simulink model "PIL_NO_RPI_new"  (R2021a)
settings: Solver=FixedStepAuto  StartTime=0.0  StopTime=60  FixedStep=0.001  RelTol=1e-3  EnableMultiTasking=on
values from neighbouring files (symbols this model uses):
  den_lpf_d = den_lpf20    [Mainframe_init.m]    (also in load_autopilot.m)
  Enable_Gyros = 0    [Mainframe_init.m]
  Enable_INS = 0    [Mainframe_init.m]
  num_lpf_d = num_lpf20    [Mainframe_init.m]    (also in load_autopilot.m)
undefined symbols (not defined in the file or in its folder): act_dmp, act_omega, Actuator, Aerodynamics, aMode, Autopilot, AUX, c_b_WGS, c_be, c_flat, c_grav, c_h_geop0, c_h_geope, c_pa0, c_pe, c_r0, c_rot, c_rsma, c_Tmp0, d_siB_0, d_siB_max, d_siB_min, dd_siB_max, dd_siB_min, dev, DiscIntNeverNeededParam, e_pa, e_Tmp, fin_maxrate, flag_I_act_switch, flag_I_aero_switch, flag_I_flat, flag_I_gravity_switch, flag_I_rot, h_bkpts_m, hcr, HIL_Data, JMMM_0, JMMM_e, JSPB_e, Ki_phi_vec, Kp_p_vec, Kp_phi_vec, lat_0, lon_0, Mass_Props, mB_0, mM_0, mM_e, National_Instruments, Newton, p, pBII_0, PCIe, phi, pMPB, pNPB, propellant_kg, prp_FBPB, prp_mdot ... (+40)
libraries: simulink x32, simulink_extras x23, aerolibcommonsys x4, pil_lib x2, custom_blocks x1, px4lib x1, sldrtlib x1, aerolibnav x1
(part 3 of 16)

== system PIL_NO_RPI_new/Non-linear Flight Dynamic Model1/Subsystem1/Extract States ==
  airfr_bus : Inport
  Assemble_States_Bus1 : Subsystem
  Bus Selector1 : BusSelector  OutputSignals=flight_dyn_bus.vBIB,flight_dyn_bus.wBIB,flight_dyn_bus.aBIB,flight_dyn_bus.d_wBIB,flight_dyn_bus.qIB,flight_dyn_bus.pBII,flight_dyn_bus.vBII
  MATLAB Function1 : MATLAB Function  TreatAsAtomicUnit=on
  quaternion_to_euler_angles1 : Subsystem
      mask help: transforms quaternions to Euler angles (roll, pitch, yaw)
      mask Help:
      | Name:
      | 
      |     quaternion_to_euler_angles
      | 
      | Description:
      | 
      |     This block implements the transformation of a quaternion into the
      |     corresponding Euler angles (zyx-sequence, roll, pitch, yaw).
      | 
      | Inputs  [size] [data type] [unit]:
      | 
      |     quaternion  [4] [double] [-]
      | 
      | Outputs  [size] [data type] [unit]:
      | 
      |     roll angle phi  [1] [double] [rad]
      |     pitch angle theta  [1] [double] [rad]
      |     yaw angle psi  [1] [double] [rad]
      mask Display:
      | %disp (' q --> (Phi,Theta,Psi) [rad]')
      | disp('q \rightarrow eu(\Phi;\Theta;\Psi)','texmode','on')
  States : Outport
  wires:
  Bus Selector1/6 -> Assemble_States_Bus1/6(POS_NED)  "<pBII>"
  quaternion_to_euler_angles1/1(eulx) -> Assemble_States_Bus1/5(Attitude_States)  "from Quat"
  MATLAB Function1/1(q_conj) -> quaternion_to_euler_angles1/1(q)
  Bus Selector1/5 -> MATLAB Function1/1(q)  "<qIB>"
  airfr_bus/1 -> Bus Selector1/1
  Bus Selector1/1 -> Assemble_States_Bus1/1(Translation_States)  "<vBIB>"
  Bus Selector1/2 -> Assemble_States_Bus1/2(Rotation_States)  "<wBIB>"
  Bus Selector1/4 -> Assemble_States_Bus1/4(Rotation_States_Dot)  "<d_wBIB>"
  Bus Selector1/3 -> Assemble_States_Bus1/3(Translation_States_Dot)  "<aBIB>"
  Assemble_States_Bus1/1(States) -> States/1
  Bus Selector1/7 -> Assemble_States_Bus1/7(POS_NED_dot)  "<vBII>"

== system PIL_NO_RPI_new/Non-linear Flight Dynamic Model1/Subsystem1/Fin Deflections ==
  Servo Deflections : Inport
  Add : Sum
  Bus Selector : BusSelector  OutputSignals=Fin_1,Fin_2,Fin_3,Fin_4
  Constant1 : Constant  Value=unc_fin_def_roll
  Constant2 : Constant  Value=unc_fin_def_pitch
  Constant3 : Constant  Value=unc_fin_def_yaw
  Degrees to Radians : Subsystem  mask(DegreesToRadians){}
      mask help: SimulinkBlocks:simulink_extras:DegreesToRadians_MD
      mask Help: web([docroot '/simulink/ref_extras/degreestoradians.html'])
      mask Display: disp('D2R')
  Degrees to Radians1 : Subsystem  mask(DegreesToRadians){}
      mask help: SimulinkBlocks:simulink_extras:DegreesToRadians_MD
      mask Help: web([docroot '/simulink/ref_extras/degreestoradians.html'])
      mask Display: disp('D2R')
  Degrees to Radians2 : Subsystem  mask(DegreesToRadians){}
      mask help: SimulinkBlocks:simulink_extras:DegreesToRadians_MD
      mask Help: web([docroot '/simulink/ref_extras/degreestoradians.html'])
      mask Display: disp('D2R')
  Vector Concatenate : Concatenate  NumInputs=4
  Vector Concatenate1 : Concatenate  NumInputs=3
  control_allocation : Subsystem
  afinB : Outport
  wires:
  Degrees to Radians2/1(Radians out) -> Vector Concatenate1/3
  Vector Concatenate1/1 -> control_allocation/1(fin_cmd)  "fin_cmd"
  Constant1/1 -> Degrees to Radians/1(Degrees in)  "xi_cmd"
  Degrees to Radians1/1(Radians out) -> Vector Concatenate1/2
  Degrees to Radians/1(Radians out) -> Vector Concatenate1/1
  Constant3/1 -> Degrees to Radians2/1(Degrees in)  "ze_cmd"
  Constant2/1 -> Degrees to Radians1/1(Degrees in)  "et_cmd"
  Bus Selector/2 -> Vector Concatenate/2  "<Fin_2>"
  Servo Deflections/1 -> Bus Selector/1
  Bus Selector/1 -> Vector Concatenate/1  "<Fin_1>"
  Bus Selector/4 -> Vector Concatenate/4  "<Fin_4>"
  Vector Concatenate/1 -> Add/1
  Bus Selector/3 -> Vector Concatenate/3  "<Fin_3>"
  control_allocation/1(siB_cmd) -> Add/2
  Add/1 -> afinB/1  "siB_cmd"

== system PIL_NO_RPI_new/Non-linear Flight Dynamic Model1/Subsystem1/GRM_Airframe ==
  siB_cmd : Inport
  T_sim_glbl : Inport  Port=2
  Bus Creator : BusCreator  Inputs=9
  aerodynamics : Subsystem
  environment : Subsystem
  fin_actuators : Subsystem
  forces_moments : Subsystem
  gravity : Subsystem
  input : Subsystem
  motion_kinematics : Subsystem
  propulsion : Subsystem
  rb_eom : Subsystem
  stream_flow : Subsystem
  weight_and_balance : Subsystem
  airfr : Outport  VectorParamsAs1DForOutWhenUnconnected=off
  wires:
  forces_moments/1(for_mom_bus) -> rb_eom/2(for_mom)
  [env] -> Bus Creator/9
  [fin] -> Bus Creator/7
  [motion_kin] -> Bus Creator/6
  [env_glbl] -> aerodynamics/4(env_glbl)
  aerodynamics/1(aero) -> forces_moments/1(aero), [aero]
  [motion_kin] -> rb_eom/1(mot_kin)
  weight_and_balance/1(wab) -> rb_eom/3(wab), gravity/2(wab), [wab], propulsion/2(wab)
  [wab] -> aerodynamics/3(wab)
  [str_flow] -> Bus Creator/5
  [motion_kin] -> forces_moments/2(motion_kin)
  motion_kinematics/1(motion_kin) -> stream_flow/2(motion_kin), [motion_kin]
  [grav] -> Bus Creator/3
  Bus Creator/1 -> airfr/1  "airfr_bus"
  [aero] -> Bus Creator/4
  environment/1(env) -> [env], stream_flow/3(env), gravity/1(env)
  [prp] -> forces_moments/4(prp)
  [prp] -> Bus Creator/8
  stream_flow/1(str_flow) -> [str_flow], aerodynamics/1(str_flow)
  input/1(cmd_bus) -> fin_actuators/1(cmd)
  [wab] -> Bus Creator/2
  gravity/1(grav) -> [grav], forces_moments/3(grav)
  T_sim_glbl/1 -> [env_glbl], environment/2(env_glbl), weight_and_balance/1(env_glb), propulsion/1(env_glbl)
  siB_cmd/1 -> input/1(siB_cmd)
  rb_eom/1(flight_dyn) -> environment/1(flight_dyn), motion_kinematics/1(flight_dyn), stream_flow/1(flight_dyn), Bus Creator/1
  fin_actuators/1(fin) -> [fin], aerodynamics/2(fin)
  propulsion/1(prp) -> [prp]

== system PIL_NO_RPI_new/Non-linear Flight Dynamic Model1/Translate Fins/Degrees to Radians ==
  Degrees in : Inport
  Gain1 : Gain  Gain=pi/180  SaturateOnIntegerOverflow=on  OutDataTypeStr=Inherit: Same as input  ParamDataTypeStr=Inherit: Same as input
  Radians out : Outport  InitialOutput=0  VectorParamsAs1DForOutWhenUnconnected=off
  wires:
  Gain1/1 -> Radians out/1
  Degrees in/1 -> Gain1/1

== system PIL_NO_RPI_new/Non-linear Flight Dynamic Model1/Translate Fins/Degrees to Radians1 ==
  Degrees in : Inport
  Gain1 : Gain  Gain=pi/180  SaturateOnIntegerOverflow=on  OutDataTypeStr=Inherit: Same as input  ParamDataTypeStr=Inherit: Same as input
  Radians out : Outport  InitialOutput=0  VectorParamsAs1DForOutWhenUnconnected=off
  wires:
  Gain1/1 -> Radians out/1
  Degrees in/1 -> Gain1/1

== system PIL_NO_RPI_new/Non-linear Flight Dynamic Model1/Translate Fins/Degrees to Radians2 ==
  Degrees in : Inport
  Gain1 : Gain  Gain=pi/180  SaturateOnIntegerOverflow=on  OutDataTypeStr=Inherit: Same as input  ParamDataTypeStr=Inherit: Same as input
  Radians out : Outport  InitialOutput=0  VectorParamsAs1DForOutWhenUnconnected=off
  wires:
  Gain1/1 -> Radians out/1
  Degrees in/1 -> Gain1/1

== system PIL_NO_RPI_new/Non-linear Flight Dynamic Model1/Translate Fins/control_allocation ==
  fin_cmd : Inport
  Constant7 : Constant  Value=Tr4r3
  Product : Product  Multiplication=Matrix(*)
  siB_cmd : Outport  VectorParamsAs1DForOutWhenUnconnected=off
  wires:
  Product/1 -> siB_cmd/1  "siB_cmd"
  fin_cmd/1 -> Product/2
  Constant7/1 -> Product/1

== system PIL_NO_RPI_new/Servos1/Real Servos/Reset Encoders ==
  Reset Encoders : Inport
  Encoder Readings : Inport  Port=2
  NOT : Logic  Operator=NOT  IconShape=distinctive  AllPortsSameDT=off  OutDataTypeStr=boolean
  Sum : Sum  Inputs=-+|
  Triggered Subsystem : Subsystem  TreatAsAtomicUnit=on
  Fin Angles : Outport
  wires:
  Encoder Readings/1 -> Sum/2, Triggered Subsystem/1(In1)
  Triggered Subsystem/1(Out1) -> Sum/1
  Reset Encoders/1 -> NOT/1
  Sum/1 -> Fin Angles/1
  NOT/1 -> Triggered Subsystem/Enable

== system PIL_NO_RPI_new/Flight Control Computer1/PixBlock/Emulated Pixhawk1/Autopilot ==
  Cmd : Inport
  IMU Data : Inport  Port=2
  INS Data : Inport  Port=3
  Bus Creator3 : BusCreator  Inputs=3
  Bus Selector : BusSelector  OutputSignals=phi_cmd
  Bus Selector1 : BusSelector  OutputSignals=gyro_x
  Bus Selector2 : BusSelector  OutputSignals=phi,z,p
  Calculate U : Subsystem
  Discrete Transfer Fcn : DiscreteTransferFcn  Numerator=[num_lpf_d]  Denominator=[den_lpf_d]
  Gain : Gain  Gain=-1
  Manual Switch : ManualSwitch
  Phi_Control : Subsystem
  Zero : Constant  Value=0  OutDataTypeStr=Inherit: Inherit via back propagation
  Attitude_Commands : Outport  VectorParamsAs1DForOutWhenUnconnected=off
  wires:
  Bus Selector1/1 -> Discrete Transfer Fcn/1  "<gyro_x>"
  IMU Data/1 -> Bus Selector1/1
  Calculate U/1(U) -> Phi_Control/5(V_mps)
  Zero/1 -> [Delta_Cmd_Psi], [Delta_Cmd_Theta]
  [Delta_Cmd_Phi] -> Bus Creator3/1  "Phi_Cmd_rad"
  [Delta_Cmd_Theta] -> Bus Creator3/2  "Theta_Cmd_rad"
  Bus Creator3/1 -> Attitude_Commands/1
  [Delta_Cmd_Psi] -> Bus Creator3/3  "Psi_Cmd_rad"
  Bus Selector/1 -> Phi_Control/1(phi_cmd_rad)  "<phi_cmd>"
  Cmd/1 -> Bus Selector/1
  INS Data/1 -> Calculate U/1(INS Data), Bus Selector2/1
  Bus Selector2/1 -> Phi_Control/2(phi_rad)  "<phi>"
  [rst] -> Phi_Control/4(Reset Integrators)
  Bus Selector2/2 -> Gain/1  "<z>"
  Gain/1 -> Phi_Control/6(h_m)
  Phi_Control/1(dela_cmd_rad) -> [Delta_Cmd_Phi]  "Phi_Cmd_rad"
  Discrete Transfer Fcn/1 -> Manual Switch/1
  Bus Selector2/3 -> Manual Switch/2  "<p>"
  Manual Switch/1 -> Phi_Control/3(p_rps)

== system PIL_NO_RPI_new/Flight Control Computer1/PixBlock/Emulated Pixhawk1/Convert to Bus ==
  Input : Inport  OutDataTypeStr=single
  100Hz Reset : Subsystem
  Bus Creator1 : BusCreator  Inputs=6
  Bus Creator2 : BusCreator  Inputs=12
  Bus Creator3 : BusCreator  Inputs=1
  Demux : Demux  Outputs=23
  Heartbeat : Outport  InitialOutput=0
  Ext. Commands : Outport  Port=2  OutDataTypeStr=single  InitialOutput=0
  Enable INS Flag : Outport  Port=3  InitialOutput=0
  Missile States : Outport  Port=4  OutDataTypeStr=single  InitialOutput=[0 0 0 0 0 0 0 0 0 0]
  Real Gyros Flag : Outport  Port=5  InitialOutput=0
  Virtual IMU Data : Outport  Port=6  OutDataTypeStr=single  InitialOutput=[0 0 0 0 0 0 0 0 0 0]
  tag scope: FCC_Enable=global, rst=global
  wires:
  Demux/22 -> Bus Creator2/12  "psi"
  Demux/21 -> Bus Creator2/11  "theta"
  Demux/20 -> Bus Creator2/10  "phi"
  Demux/4 -> Real Gyros Flag/1  "Real Gyros Flag"
  Demux/5 -> Bus Creator2/1  "u"
  Demux/18 -> Bus Creator1/5  "gyro_y"
  Bus Creator1/1 -> Virtual IMU Data/1
  Demux/16 -> Bus Creator1/3  "acc_z"
  Demux/9 -> Bus Creator2/5  "y"
  Demux/14 -> Bus Creator1/1  "acc_x"
  Demux/17 -> Bus Creator1/4  "gyro_x"
  Demux/15 -> Bus Creator1/2  "acc_y"
  Demux/19 -> Bus Creator1/6  "gyro_z"
  Demux/12 -> Bus Creator2/8  "q"
  Demux/7 -> Bus Creator2/3  "w"
  Demux/10 -> Bus Creator2/6  "z"
  Demux/6 -> Bus Creator2/2  "v"
  Demux/11 -> Bus Creator2/7  "p"
  Demux/13 -> Bus Creator2/9  "r"
  Demux/23 -> Bus Creator3/1  "phi_cmd"
  Demux/8 -> Bus Creator2/4  "x"
  Bus Creator3/1 -> Ext. Commands/1
  Bus Creator2/1 -> Missile States/1
  Demux/1 -> [FCC_Enable]  "EnableFCC"
  Input/1 -> Demux/1
  Demux/2 -> 100Hz Reset/1(Heartbeat), Heartbeat/1  "Hearbeat"
  Demux/3 -> Enable INS Flag/1  "Enable INS Flag"
  100Hz Reset/1(RST) -> [rst]

== system PIL_NO_RPI_new/Flight Control Computer1/PixBlock/Emulated Pixhawk1/Convert to Vector ==
  Fin Deflections : Inport
  Heartbeat : Inport  Port=2
  INS Data : Inport  Port=3
  Real Gyro Data : Inport  Port=4
  Debug Port : Inport  Port=5
  Bus Selector1 : BusSelector  OutputSignals=Fin_1_Cmd_rad,Fin_2_Cmd_rad,Fin_3_Cmd_rad,Fin_4_Cmd_rad
  Bus Selector2 : BusSelector  OutputSignals=gyro_x,gyro_y,gyro_z
  Bus Selector3 : BusSelector  OutputSignals=u,v,w,x,y,z,p,q,r
  Cast To Single : DataTypeConversion  OutDataTypeStr=single
  Vector Concatenate : Concatenate  NumInputs=18
  To HIL : Outport
  wires:
  Bus Selector1/3 -> Vector Concatenate/4  "<Fin_3_Cmd_rad>"
  Bus Selector1/4 -> Vector Concatenate/5  "<Fin_4_Cmd_rad>"
  Heartbeat/1 -> Vector Concatenate/1
  Bus Selector1/1 -> Vector Concatenate/2  "<Fin_1_Cmd_rad>"
  Bus Selector1/2 -> Vector Concatenate/3  "<Fin_2_Cmd_rad>"
  Vector Concatenate/1 -> Cast To Single/1
  Fin Deflections/1 -> Bus Selector1/1
  Cast To Single/1 -> To HIL/1
  Real Gyro Data/1 -> Bus Selector2/1
  Bus Selector3/7 -> Vector Concatenate/15  "<p>"
  Bus Selector3/5 -> Vector Concatenate/13  "<y>"
  Bus Selector3/4 -> Vector Concatenate/12  "<x>"
  Bus Selector3/9 -> Vector Concatenate/17  "<r>"
  Bus Selector3/3 -> Vector Concatenate/11  "<w>"
  Bus Selector2/3 -> Vector Concatenate/8  "<gyro_z>"
  Debug Port/1 -> Vector Concatenate/18
  Bus Selector3/1 -> Vector Concatenate/9  "<u>"
  Bus Selector2/2 -> Vector Concatenate/7  "<gyro_y>"
  Bus Selector2/1 -> Vector Concatenate/6  "<gyro_x>"
  Bus Selector3/8 -> Vector Concatenate/16  "<q>"
  INS Data/1 -> Bus Selector3/1
  Bus Selector3/6 -> Vector Concatenate/14  "<z>"
  Bus Selector3/2 -> Vector Concatenate/10  "<v>"

== system PIL_NO_RPI_new/Flight Control Computer1/PixBlock/Emulated Pixhawk1/Fin Allocation ==
  Attitude Cmd : Inport
  Bus Creator : BusCreator  Inputs=4
  Bus Selector : BusSelector  OutputSignals=Phi_Cmd_rad,Theta_Cmd_rad,Psi_Cmd_rad
  Demux : Demux
  Vector Concatenate1 : Concatenate  NumInputs=3
  control_allocation : Subsystem
  Fin Cmd : Outport  VectorParamsAs1DForOutWhenUnconnected=off
  wires:
  Demux/4 -> Bus Creator/4  "Fin_4_Cmd_rad"
  control_allocation/1(siB_cmd) -> Demux/1
  Bus Selector/3 -> Vector Concatenate1/3  "<Psi_Cmd_rad>"
  Vector Concatenate1/1 -> control_allocation/1(fin_cmd)  "fin_cmd"
  Bus Selector/1 -> Vector Concatenate1/1  "<Phi_Cmd_rad>"
  Demux/3 -> Bus Creator/3  "Fin_3_Cmd_rad"
  Bus Selector/2 -> Vector Concatenate1/2  "<Theta_Cmd_rad>"
  Demux/1 -> Bus Creator/1  "Fin_1_Cmd_rad"
  Bus Creator/1 -> Fin Cmd/1
  Attitude Cmd/1 -> Bus Selector/1
  Demux/2 -> Bus Creator/2  "Fin_2_Cmd_rad"

== system PIL_NO_RPI_new/Flight Control Computer1/PixBlock/Emulated Pixhawk1/IMU - Merge ==
  HIL IMU : Inport
  Bus Creator2 : BusCreator  Inputs=6
  Bus Selector2 : BusSelector  OutputSignals=acc_x,acc_y,acc_z,gyro_x,gyro_y,gyro_z
  IMU Data : Outport
  wires:
  HIL IMU/1 -> Bus Selector2/1
  Bus Selector2/5 -> Bus Creator2/5  "<gyro_y>"
  Bus Selector2/6 -> Bus Creator2/6  "<gyro_z>"
  Bus Selector2/4 -> Bus Creator2/4  "<gyro_x>"
  Bus Selector2/2 -> Bus Creator2/2  "<acc_y>"
  Bus Selector2/1 -> Bus Creator2/1  "<acc_x>"
  Bus Selector2/3 -> Bus Creator2/3  "<acc_z>"
  Bus Creator2/1 -> IMU Data/1

== system PIL_NO_RPI_new/Flight Control Computer1/PixBlock/Emulated Pixhawk1/Inertial Navigation System ==
  Enable INS Flag : Inport
  Missile States : Inport  Port=2
  IMU Data : Inport  Port=3
  INS (INCOMPLETE) : Subsystem
  Switch : Switch  Criteria=u2 > Threshold
  INS Data : Outport
  wires:
  Enable INS Flag/1 -> Switch/2
  IMU Data/1 -> INS (INCOMPLETE)/1(IMU Data)
  Switch/1 -> INS Data/1
  Missile States/1 -> Switch/3
  INS (INCOMPLETE)/1(INS Data) -> Switch/1

== system PIL_NO_RPI_new/Flight Control Computer1/PixBlock/Emulated Pixhawk1/Real Gyro ==
  HIL Gyro : Inport
  Bus Creator2 : BusCreator  Inputs=3
  Bus Selector2 : BusSelector  OutputSignals=gyro_x,gyro_y,gyro_z
  Gyro Data : Outport
  wires:
  HIL Gyro/1 -> Bus Selector2/1
  Bus Selector2/2 -> Bus Creator2/2  "<gyro_y>"
  Bus Selector2/1 -> Bus Creator2/1  "<gyro_x>"
  Bus Selector2/3 -> Bus Creator2/3  "<gyro_z>"
  Bus Creator2/1 -> Gyro Data/1

== system PIL_NO_RPI_new/Flight Control Computer1/PixBlock/Emulated Pixhawk1/Servo Commands ==
  Fin Cmd : Inport
  100Hz Progress : Subsystem
  AND : Logic  IconShape=distinctive  AllPortsSameDT=off  OutDataTypeStr=boolean
  Add{,1..3} (4 alike) : Sum
  Bus Selector : BusSelector  OutputSignals=Fin_1_Cmd_rad,Fin_2_Cmd_rad,Fin_3_Cmd_rad,Fin_4_Cmd_rad
  Cast To Boolean : DataTypeConversion  OutDataTypeStr=boolean
  Cast To Double{,1..3} (4 alike) : DataTypeConversion  OutDataTypeStr=uint16
  Gain{,1..3} (4 alike) : Gain  Gain=1000/91
  One{,1..3} (4 alike) : Constant  Value=1500  OutDataTypeStr=Inherit: Inherit via back propagation
  One4 : Constant  Value=0  OutDataTypeStr=boolean
  PX4 PWM Output1 : px4lib/PX4 PWM Output  pwmDevice=AUX (/dev/pwm_output1)  pwmChannel1_=on  pwmChannel2_=on  pwmChannel3_=on  pwmChannel4_=on  pwmChannel5_=off  pwmChannel6_=off  pwmChannel7_=off  pwmChannel8_=off  forceTerminateFailsafe=off  outputErrorStatus=off
      settings: SourceProductBaseCode=PX4AUTOPILOTS
  Radians to Degrees{,1..3} (4 alike) : simulink_extras/Transformations/Radians to Degrees
  Saturation{,1..3} (4 alike) : Saturate  UpperLimit=20  LowerLimit=-20
  wires:
  Saturation2/1 -> Gain2/1
  Cast To Double3/1 -> PX4 PWM Output1/6
  One4/1 -> PX4 PWM Output1/2
  One/1 -> Add/2
  One2/1 -> Add2/2
  Add1/1 -> Cast To Double1/1
  Gain2/1 -> Add2/1
  AND/1 -> Cast To Boolean/1
  Radians to Degrees1/1 -> Saturation1/1
  Cast To Double2/1 -> PX4 PWM Output1/5
  Add2/1 -> Cast To Double2/1
  Fin Cmd/1 -> Bus Selector/1
  Cast To Double1/1 -> PX4 PWM Output1/4
  Bus Selector/2 -> Radians to Degrees1/1  "<Fin_2_Cmd_rad>"
  Gain/1 -> Add/1
  Bus Selector/4 -> Radians to Degrees3/1  "<Fin_4_Cmd_rad>"
  One3/1 -> Add3/2
  Saturation/1 -> Gain/1
  Gain1/1 -> Add1/1
  Saturation3/1 -> Gain3/1
  Gain3/1 -> Add3/1
  Radians to Degrees3/1 -> Saturation3/1
  Bus Selector/1 -> Radians to Degrees/1  "<Fin_1_Cmd_rad>"
  Bus Selector/3 -> Radians to Degrees2/1  "<Fin_3_Cmd_rad>"
  Saturation1/1 -> Gain1/1
  Cast To Double/1 -> PX4 PWM Output1/3
  Add3/1 -> Cast To Double3/1
  Radians to Degrees2/1 -> Saturation2/1
  [FCC_Enable] -> AND/1
  Radians to Degrees/1 -> Saturation/1
  100Hz Progress/1(RST) -> AND/2
  One1/1 -> Add1/2
  Add/1 -> Cast To Double/1
  Cast To Boolean/1 -> PX4 PWM Output1/1

== system PIL_NO_RPI_new/Flight Control Computer2/Pixhawk1/FCC Logic1/Control ==
  cmd : Inport
  states : Inport  Port=2
  ALT : Inport  Port=3
  100 Hz : DiscretePulseGenerator  PulseType=Time based  Period=0.01  PulseWidth=50
  Bus Selector : BusSelector  OutputSignals=phi_cmd
  Bus Selector1 : BusSelector  OutputSignals=u,v,w
  Bus Selector2 : BusSelector  OutputSignals=phi,p
  Cast To Double32 : DataTypeConversion  OutDataTypeStr=double
  Constant1 : Constant  Value=0  SampleTime=-1
  Phi Controller : Subsystem
  Subsystem : Subsystem
  states1 : InportShadow  Port=2
  Attitude_Commands : Outport  VectorParamsAs1DForOutWhenUnconnected=off
  wires:
  Cast To Double32/1 -> Phi Controller/6(integrators_active)
  100 Hz/1 -> Phi Controller/Trigger
  cmd/1 -> Bus Selector/1
  Bus Selector2/2 -> Phi Controller/3(ps_f_rps)  "<p>"
  Bus Selector2/1 -> Phi Controller/2(phi_fb_rad)  "<phi>"
  Bus Selector/1 -> Phi Controller/1(phi_cmd_rad)  "<phi_cmd>"
  states/1 -> Bus Selector2/1
  Phi Controller/1(dela_cmd_rad) -> Attitude_Commands/1  "Phi_Cmd_rad"
  Bus Selector1/1 -> Subsystem/1(<u>)  "<u>"
  Bus Selector1/2 -> Subsystem/2(<v>)  "<v>"
  Bus Selector1/3 -> Subsystem/3(<w>)  "<w>"
  Subsystem/1(U) -> Phi Controller/4(V_mps)
  states1/1 -> Bus Selector1/1
  ALT/1 -> Phi Controller/5(h_m)
  Constant1/1 -> Cast To Double32/1

== system PIL_NO_RPI_new/Flight Control Computer2/Pixhawk1/FCC Logic1/Fin Allocation ==
  Input1 : Inport
  Constant : Constant  Value=0
  Constant1 : Constant  Value=0
  Constant2 : Constant  Value=unc_fin_def_roll
  Constant5 : Constant  Value=unc_fin_def_pitch
  Constant8 : Constant  Value=unc_fin_def_yaw
  Degrees to Radians1 : simulink_extras/Transformations/Degrees to Radians
  Degrees to Radians2 : simulink_extras/Transformations/Degrees to Radians
  Degrees to Radians3 : simulink_extras/Transformations/Degrees to Radians
  Gain1 : Gain  Gain=180/pi
      settings: AttributesFormatString=%<Gain>
  Gain2 : Gain  Gain=180/pi
      settings: AttributesFormatString=%<Gain>
  Gain3 : Gain  Gain=180/pi
      settings: AttributesFormatString=%<Gain>
  Saturation1 : Saturate  UpperLimit=20  LowerLimit=-20
  Saturation2 : Saturate  UpperLimit=20  LowerLimit=-20
  Saturation3 : Saturate  UpperLimit=20  LowerLimit=-20
  Subsystem : Subsystem  Commented=on
  Sum1 : Sum
  Sum2 : Sum
  Sum3 : Sum
  Vector Concatenate1 : Concatenate  NumInputs=3
  siB_cmd : Outport  VectorParamsAs1DForOutWhenUnconnected=off
  wires:
  Saturation2/1 -> Sum2/1
  Constant1/1 -> Gain3/1
  Saturation3/1 -> Sum3/1
  Sum1/1 -> Degrees to Radians1/1  "xi_cmd"
  Degrees to Radians2/1 -> Vector Concatenate1/2
  Degrees to Radians3/1 -> Vector Concatenate1/3
  Constant/1 -> Gain2/1
  Sum2/1 -> Degrees to Radians2/1  "et_cmd"
  Input1/1 -> Gain1/1
  Constant2/1 -> Sum1/2
  Degrees to Radians1/1 -> Vector Concatenate1/1
  Saturation1/1 -> Sum1/1
  Gain1/1 -> Saturation1/1  "dela_cmd_deg"
  Gain3/1 -> Saturation3/1  "delr_cmd_deg"
  Gain2/1 -> Saturation2/1  "dele_cmd_deg"
  Sum3/1 -> Degrees to Radians3/1  "ze_cmd"
  Constant8/1 -> Sum3/2
  Constant5/1 -> Sum2/2
  Vector Concatenate1/1 -> siB_cmd/1  "fin_cmd"

== system PIL_NO_RPI_new/Flight Control Computer2/Pixhawk1/FCC Logic1/variable switch ==
  Simulation States : Inport
  Bus Assignment : BusAssignment  AssignedSignals=p,q,r,phi,theta,psi
  Bus Selector : BusSelector  OutputSignals=p,q,r,phi,theta,psi
  State Bus : Outport
  wires:
  Simulation States/1 -> Bus Assignment/1, Bus Selector/1
  Bus Assignment/1 -> State Bus/1
  Bus Selector/1 -> Bus Assignment/2  "<p>"
  Bus Selector/2 -> Bus Assignment/3  "<q>"
  Bus Selector/3 -> Bus Assignment/4  "<r>"
  Bus Selector/4 -> Bus Assignment/5  "<phi>"
  Bus Selector/5 -> Bus Assignment/6  "<theta>"
  Bus Selector/6 -> Bus Assignment/7  "<psi>"

== system PIL_NO_RPI_new/Flight Control Computer2/Pixhawk1/Send to HIL/control_allocation1 ==
  fin_cmd : Inport
  Cast To Single1 : DataTypeConversion  OutDataTypeStr=single
  Constant7 : Constant  Value=Tr4r3
  Product : Product  Multiplication=Matrix(*)
  siB_cmd : Outport  VectorParamsAs1DForOutWhenUnconnected=off
  wires:
  Constant7/1 -> Product/1
  fin_cmd/1 -> Cast To Single1/1
  Product/1 -> siB_cmd/1  "siB_cmd"
  Cast To Single1/1 -> Product/2

== system PIL_NO_RPI_new/Flight Gear Simulator/Flight Simulator On/Flat Earth to LLA/LatLong wrap ==
  LatLong : Inport
  Constant : Constant  Value=180
  Constant1 : Constant  Value=0
  Demux : Demux  Outputs=2
  Latitude Wrap 90 : Subsystem  mask(LatitudeWrap90){}
      mask init:
      | aeroicon('aeroblk')
  Mux : Mux  Inputs=2
  Sum : Sum  Inputs=|++
  Switch1 : Switch  Criteria=u2 ~= 0
  Wrap Longitude : Subsystem
      mask init:
      | aeroicon('aeroblk');
  Lat/Long wrapped : Outport  VectorParamsAs1DForOutWhenUnconnected=off
  wires:
  Latitude Wrap 90/1(Lat wrapped) -> Mux/1
  Latitude Wrap 90/2(Wrap flag) -> Switch1/2
  Demux/1 -> Latitude Wrap 90/1(Lat)
  Wrap Longitude/1(Angle 180) -> Mux/2
  Mux/1 -> Lat/Long wrapped/1
  Sum/1 -> Wrap Longitude/1(Angle)
  Demux/2 -> Sum/2
  Switch1/1 -> Sum/1
  Constant1/1 -> Switch1/3
  Constant/1 -> Switch1/1
  LatLong/1 -> Demux/1

== system PIL_NO_RPI_new/Flight Gear Simulator/Flight Simulator On/Flat Earth to LLA/LatLong wrap1 ==
  LatLong : Inport
  Constant : Constant  Value=180
  Constant1 : Constant  Value=0
  Demux : Demux  Outputs=2
  Latitude Wrap 90 : Subsystem  mask(LatitudeWrap90){}
      mask init:
      | aeroicon('aeroblk')
  Mux : Mux  Inputs=2
  Sum : Sum  Inputs=|++
  Switch1 : Switch  Criteria=u2 ~= 0
  Wrap Longitude : Subsystem
      mask init:
      | aeroicon('aeroblk');
  Lat/Long wrapped : Outport  VectorParamsAs1DForOutWhenUnconnected=off
  wires:
  Latitude Wrap 90/1(Lat wrapped) -> Mux/1
  Latitude Wrap 90/2(Wrap flag) -> Switch1/2
  Demux/1 -> Latitude Wrap 90/1(Lat)
  Wrap Longitude/1(Angle 180) -> Mux/2
  Mux/1 -> Lat/Long wrapped/1
  Sum/1 -> Wrap Longitude/1(Angle)
  Demux/2 -> Sum/2
  Switch1/1 -> Sum/1
  Constant1/1 -> Switch1/3
  Constant/1 -> Switch1/1
  LatLong/1 -> Demux/1

== system PIL_NO_RPI_new/Flight Gear Simulator/Flight Simulator On/Flat Earth to LLA/LongLat_offset ==
  XY : Inport
  mu : Inport  Port=2
  Angle Conversion2 : Subsystem
  Demux : Demux  Outputs=2
  Find Radian/Distance : Subsystem
  Mux : Mux  Inputs=2
  SinCos : Trigonometry  Operator=sincos
  Sum : Sum  Inputs=|+-
  Sum1 : Sum  Inputs=|++
  rad lat : Product  RndMeth=Zero
  "rad long " : Product  RndMeth=Zero
  ref_pos : Constant  Value=psi
  x*cos : Product  RndMeth=Zero
  x*sin : Product  RndMeth=Zero
  y*cos : Product  RndMeth=Zero
  y*sin : Product  RndMeth=Zero
  DeltaLL_rad : Outport  VectorParamsAs1DForOutWhenUnconnected=off
  wires:
  mu/1 -> Find Radian/Distance/1(mu)
  Find Radian/Distance/1(dNorth) -> rad lat/2
  Find Radian/Distance/2(dEast) -> "rad long "/1
  rad lat/1 -> Mux/1
  "rad long "/1 -> Mux/2
  Mux/1 -> DeltaLL_rad/1
  Angle Conversion2/1(out) -> SinCos/1
  Demux/2 -> y*cos/1, y*sin/1
  Sum1/1 -> "rad long "/2
  y*cos/1 -> Sum1/2
  x*sin/1 -> Sum1/1
  Sum/1 -> rad lat/1
  y*sin/1 -> Sum/2
  SinCos/1 -> x*sin/2, y*sin/2
  x*cos/1 -> Sum/1
  SinCos/2 -> y*cos/2, x*cos/2
  Demux/1 -> x*sin/1, x*cos/1
  XY/1 -> Demux/1
  ref_pos/1 -> Angle Conversion2/1(in)

== system PIL_NO_RPI_new/Flight Gear Simulator/Flight Simulator On/Flat Earth to LLA/pos_deg ==
  in : Inport  Unit=rad
  Unit Conversion : UnitConversion
  out : Outport  Unit=deg  VectorParamsAs1DForOutWhenUnconnected=off
  wires:
  in/1 -> Unit Conversion/1
  Unit Conversion/1 -> out/1

== system PIL_NO_RPI_new/Flight Gear Simulator/Flight Simulator On/FlightGear Preconfigured 6DoF Animation/Angle Conversion ==
  in : Inport  Unit=deg
  Unit Conversion : UnitConversion
  out : Outport  Unit=rad  VectorParamsAs1DForOutWhenUnconnected=off
  wires:
  in/1 -> Unit Conversion/1
  Unit Conversion/1 -> out/1

== system PIL_NO_RPI_new/Flight Gear Simulator/Flight Simulator On/FlightGear Preconfigured 6DoF Animation/Angle Conversion1 ==
  in : Inport  Unit=deg
  Unit Conversion : UnitConversion
  out : Outport  Unit=rad  VectorParamsAs1DForOutWhenUnconnected=off
  wires:
  Unit Conversion/1 -> out/1
  in/1 -> Unit Conversion/1

== system PIL_NO_RPI_new/Non-linear Flight Dynamic Model1/Environment/atm_dynamic/trafo_around_z_axis ==
  vec1 : Inport
  gamma : Inport  Port=2
  1_rot_mat : Subsystem  mask(Rotation um 1, 2 oder 3 Achsen){rot_1=Rotation um z-Achse}
      mask prompts: rot_1 "1. Rotation"
      mask help:
      | Dieser Block liefert die Rotationsmatrix T12 für den Fall zurück, dass sich das Ziel-Koordinatensystem (1) durch Drehungen um 1, 2 oder 3 Achsen gegenüber dem Ausgangskoordinatensystem (2) beschreiben lässt (passive Drehung).
      |
      | Die Anzahl der Rotation sowie die Reihenfolge ist frei einstellbar.
      |
      | Die Rotationswinkel haben die Einheit [rad].
      mask TypeOptions rot_1: Rotation um x-Achse | Rotation um y-Achse | Rotation um z-Achse
  Product : Product  Multiplication=Matrix(*)
  Reshape : Reshape  OutputDimensionality=Column vector (2-D)
  vec2 : Outport  VectorParamsAs1DForOutWhenUnconnected=off
  wires:
  Product/1 -> vec2/1  "vec2"
  gamma/1 -> 1_rot_mat/1(wi1)  "gamma"
  1_rot_mat/1(T12) -> Product/1  "T12"
  vec1/1 -> Reshape/1  "vec1"
  Reshape/1 -> Product/2  "vec1"

== system PIL_NO_RPI_new/Non-linear Flight Dynamic Model1/Extract States/Assemble_States_Bus1/Rotation Angles to Quaternions ==
  "R1, R2, R3" : Inport  Unit=rad
  1/2 : Gain  Gain=0.5  SaturateOnIntegerOverflow=on  OutDataTypeStr=Inherit: Same as input  ParamDataTypeStr=Inherit: Same as input
  Mux1 : Mux  Inputs=2
  Mux2 : Mux
  q0 : Fcn  Expr=u(4)*u(5)*u(6) + u(1)*u(2)*u(3)
  q1 : Fcn  Expr=u(4)*u(5)*u(3) - u(1)*u(2)*u(6)
  q2 : Fcn  Expr=u(4)*u(2)*u(6) + u(1)*u(5)*u(3)
  q3 : Fcn  Expr=u(1)*u(5)*u(6) - u(4)*u(2)*u(3)
  sincos : Trigonometry  Operator=sincos
  Quat : Outport  Unit=1  InitialOutput=0  VectorParamsAs1DForOutWhenUnconnected=off
  wires:
  q0/1 -> Mux2/1
  Mux2/1 -> Quat/1
  q3/1 -> Mux2/4
  q2/1 -> Mux2/3
  q1/1 -> Mux2/2
  Mux1/1 -> q3/1, q2/1, q1/1, q0/1
  sincos/2 -> Mux1/2
  sincos/1 -> Mux1/1
  1/2/1 -> sincos/1
  "R1, R2, R3"/1 -> 1/2/1

== system PIL_NO_RPI_new/Non-linear Flight Dynamic Model1/Extract States/Assemble_States_Bus1/Three-axis Inertial Measurement Unit3 ==
  A_b : Inport  Unit=m/s^2
  w : Inport  Port=2  Unit=rad/s
  w_dot : Inport  Port=3  Unit=rad/s^2
  CG : Inport  Port=4  Unit=m
  g : Inport  Port=5  Unit=m/s^2
  Acceleration Conversion : Subsystem
  Disallow CGS : UnitConfiguration  UnitSystemsStr=English,SI,SI (extended)  AllowAllUnitSystems=off
  Three-axis Accelerometer : Subsystem  mask(Three-axis Accelerometer){units=Metric (MKS), acc=imu, gtype=on, dtype_a=on, w_a=w_a, z_a=z_a, a_sf_cc=a_sf_cc, a_bias=a_bias, a_Ts=i_Ts, a_rand=on, a_seeds=i_seeds(1:3), a_pow=i_pow(1:3), a_sat=a_sat}
      mask prompts: units "aeroblks:aeroblknav:blockThreeaxisAccelerometerParamUnits"; acc "aeroblks:aeroblknav:blockThreeaxisAccelerometerParamAccelerometerlocation"; gtype "aeroblks:aeroblknav:blockThreeaxisAccelerometerParamSubtractgravity"; dtype_a "aeroblks:aeroblknav:blockThreeaxisAccelerometerParamSecondorderdynamics"; w_a "aeroblks:aeroblknav:blockThreeaxisAccelerometerParamNaturalfrequencyradsec"; z_a "aeroblks:aeroblknav:blockThreeaxisAccelerometerParamDampingratio"; a_sf_cc "aeroblks:aeroblknav:blockThreeaxisAccelerometerParamScalefactorsandcrosscoupling"; a_bias "aeroblks:aeroblknav:blockThreeaxisAccelerometerParamMeasurementbias"; a_Ts "aeroblks:aeroblknav:blockThreeaxisAccelerometerParamUpdateratesec"; a_rand "aeroblks:aeroblknav:blockThreeaxisAccelerometerParamNoiseon"; a_seeds "aeroblks:aeroblknav:blockThreeaxisAccelerometerParamNoiseseeds"; a_pow "aeroblks:aeroblknav:blockThreeaxisAccelerometerParamNoisepower"; a_sat "aeroblks:aeroblknav:blockThreeaxisAccelerometerParamLowerandupperoutputlimits"
      mask help: aeroblks:aeroblknav:blockThreeaxisAccelerometerDesc
      mask init:
      | par = a_Ts;
      | block = gcb;
      | ports=aeroicon('aeroblkaccel','icon',par);
      | a_satl = a_sat(1:3);
      | a_sath = a_sat(4:6);
      mask Help: eval('asbhelp');
      mask TypeOptions units: aeroblks:aeroblknav:blockThreeaxisAccelerometerParamComboMetricMKS | aeroblks:aeroblknav:blockThreeaxisAccelerometerParamComboEnglish
      mask Callback gtype: aeroicon('aeroblkaccel')
      mask Callback dtype_a: aeroicon('aeroblkaccel')
      mask Callback a_rand: aeroicon('aeroblkaccel')
      mask DialogControl ParameterTabVar0 Prompt: Main
      mask DialogControl units Prompt: Units:
      mask DialogControl acc Prompt: Accelerometer location:
      mask DialogControl gtype Prompt: Subtract gravity:
      mask DialogControl dtype_a Prompt: Second-order dynamics
      mask DialogControl w_a Prompt: Natural frequency (rad/sec):
      mask DialogControl z_a Prompt: Damping ratio:
      mask DialogControl a_sf_cc Prompt: Scale factors and cross-coupling:
      mask DialogControl a_bias Prompt: Measurement bias:
      mask DialogControl a_Ts Prompt: Update rate (sec):
      mask DialogControl ParameterTabVar01 Prompt: Noise
      mask DialogControl a_rand Prompt: Noise on
      mask DialogControl a_seeds Prompt: Noise seeds:
      mask DialogControl a_pow Prompt: Noise power:
      mask DialogControl a_sat Prompt: Lower and upper output limits:
      mask Display:
      | port_label(ports(1).type,ports(1).port,ports(1).txt,'texmode','on');
      | port_label(ports(2).type,ports(2).port,ports(2).txt,'texmode','on');
      | port_label(ports(3).type,ports(3).port,ports(3).txt,'texmode','on');
      | port_label(ports(4).type,ports(4).port,ports(4).txt,'texmode','on');
      | port_label(ports(5).type,ports(5).port,ports(5).txt,'texmode','on');
      | port_label(ports(6).type,ports(6).port,ports(6).txt,'texmode','on');
  Three-axis Gyroscope : Subsystem  mask(Three-axis Gyroscope){dtype_g=on, w_g=w_g, z_g=z_g, g_sf_cc=g_sf_cc, g_bias=g_bias, g_sen=g_sens, g_Ts=i_Ts, g_rand=on, g_seeds=i_seeds(4:6), g_pow=i_pow(4:6), g_sat=g_sat}
      mask prompts: dtype_g "aeroblks:aeroblknav:blockThreeaxisGyroscopeParamSecondorderdynamics"; w_g "aeroblks:aeroblknav:blockThreeaxisGyroscopeParamNaturalfrequencyradsec"; z_g "aeroblks:aeroblknav:blockThreeaxisGyroscopeParamDampingratio"; g_sf_cc "aeroblks:aeroblknav:blockThreeaxisGyroscopeParamScalefactorsandcrosscoupling"; g_bias "aeroblks:aeroblknav:blockThreeaxisGyroscopeParamMeasurementbias"; g_sen "aeroblks:aeroblknav:blockThreeaxisGyroscopeParamGsensitivebias"; g_Ts "aeroblks:aeroblknav:blockThreeaxisGyroscopeParamUpdateratesec"; g_rand "aeroblks:aeroblknav:blockThreeaxisGyroscopeParamNoiseon"; g_seeds "aeroblks:aeroblknav:blockThreeaxisGyroscopeParamNoiseseeds"; g_pow "aeroblks:aeroblknav:blockThreeaxisGyroscopeParamNoisepower"; g_sat "aeroblks:aeroblknav:blockThreeaxisGyroscopeParamLowerandupperoutputlimits"
      mask help: aeroblks:aeroblknav:blockThreeaxisGyroscopeDesc
      mask init:
      | par = g_Ts;
      | block = gcb;
      | g_satl = g_sat(1:3);
      | g_sath = g_sat(4:6);
      | ports=aeroicon('aeroblkgyro','icon',par);
      mask Help: eval('asbhelp');
      mask Callback dtype_g: aeroicon('aeroblkgyro');
      mask Callback g_rand: aeroicon('aeroblkgyro');
      mask DialogControl ParameterTabVar0 Prompt: Main
      mask DialogControl dtype_g Prompt: Second-order dynamics
      mask DialogControl w_g Prompt: Natural frequency (rad/sec):
      mask DialogControl z_g Prompt: Damping ratio:
      mask DialogControl g_sf_cc Prompt: Scale factors and cross-coupling:
      mask DialogControl g_bias Prompt: Measurement bias:
      mask DialogControl g_sen Prompt: G-sensitive bias:
      mask DialogControl g_Ts Prompt: Update rate (sec):
      mask DialogControl ParameterTabVar01 Prompt: Noise
      mask DialogControl g_rand Prompt: Noise on
      mask DialogControl g_seeds Prompt: Noise seeds:
      mask DialogControl g_pow Prompt: Noise power:
      mask DialogControl g_sat Prompt: Lower and upper output limits:
      mask Display:
      | port_label(ports(1).type,ports(1).port,ports(1).txt,'texmode','on');
      | port_label(ports(2).type,ports(2).port,ports(2).txt,'texmode','on');
      | port_label(ports(3).type,ports(3).port,ports(3).txt,'texmode','on');
  A_meas : Outport  Unit=m/s^2  VectorParamsAs1DForOutWhenUnconnected=off
  w_meas : Outport  Port=2  Unit=rad/s  VectorParamsAs1DForOutWhenUnconnected=off
  wires:
  Three-axis Accelerometer/1(Ameas) -> A_meas/1
  Three-axis Gyroscope/1((p q r)_meas) -> w_meas/1
  A_b/1 -> Acceleration Conversion/1(acceleration), Three-axis Accelerometer/1(Ab)
  w/1 -> Three-axis Accelerometer/2(p q r), Three-axis Gyroscope/1(p q r)
  CG/1 -> Three-axis Accelerometer/4(CG)
  w_dot/1 -> Three-axis Accelerometer/3(pdot qdot rdot)
  Acceleration Conversion/1(inherit) -> Three-axis Gyroscope/2(G's)
  g/1 -> Three-axis Accelerometer/5(g)

== system PIL_NO_RPI_new/Non-linear Flight Dynamic Model1/GRM_Airframe/aerodynamics/aerodynamic_via_lookup ==
  pBPB : Inport
  qdynB : Inport  Port=2
  MaB : Inport  Port=3
  alB : Inport  Port=4
  beB : Inport  Port=5
  hBE : Inport  Port=6
  wBIB_star : Inport  Port=7
  afinB : Inport  Port=8
  flag_I_prp : Inport  Port=9
  Bus Creator : BusCreator  Inputs=2
  Demux1 : Demux  Outputs=3
  Demux3 : Demux  Outputs=3
  Gain{,1..4} (5 alike) : Gain  Gain=180/pi
      settings: AttributesFormatString=%<Gain>
  Saturation1 : Saturate  UpperLimit=Aerodynamics.ulim_alpha_deg  LowerLimit=Aerodynamics.llim_alpha_deg
      settings: AttributesFormatString=|
      | %<UpperLimit>
      | %<LowerLimit>
  Saturation4 : Saturate  UpperLimit=Aerodynamics.ulim_beta_deg  LowerLimit=Aerodynamics.llim_beta_deg
      settings: AttributesFormatString=|
      | %<UpperLimit>
      | %<LowerLimit>
  Terminator : Terminator
  Terminator1 : Terminator
  calc_aero_coefficients : Subsystem
  calc_aero_for_mom : Subsystem
  aero_bus : Outport  VectorParamsAs1DForOutWhenUnconnected=off
  wires:
  MaB/1 -> Terminator1/1
  calc_aero_for_mom/1(FBAB) -> Bus Creator/1
  Bus Creator/1 -> aero_bus/1  "aero_bus"
  pBPB/1 -> calc_aero_for_mom/2(pBPB)
  flag_I_prp/1 -> Terminator/1
  hBE/1 -> calc_aero_for_mom/1(hBE)
  calc_aero_for_mom/2(MBAB) -> Bus Creator/2
  qdynB/1 -> calc_aero_for_mom/3(qdynB)
  alB/1 -> Gain3/1
  beB/1 -> Gain4/1
  wBIB_star/1 -> Demux1/1
  Demux1/1 -> calc_aero_coefficients/4(pBIB_star_rps)  "pBIB_star_rps"
  Demux1/2 -> calc_aero_coefficients/5(qBIB_star_rps)  "qBIB_star_rps"
  Demux1/3 -> calc_aero_coefficients/6(rBIB_star_rps)  "rBIB_star_rps"
  afinB/1 -> Demux3/1
  Demux3/2 -> Gain1/1  "etB"
  Demux3/1 -> Gain/1  "xiB"
  Demux3/3 -> Gain2/1  "zeB"
  Gain/1 -> calc_aero_coefficients/1(dela_deg)
  Gain1/1 -> calc_aero_coefficients/2(dele_deg)
  Gain2/1 -> calc_aero_coefficients/3(delr_deg)
  calc_aero_coefficients/1(Cx) -> calc_aero_for_mom/4(Cx)
  calc_aero_coefficients/2(Cy) -> calc_aero_for_mom/5(Cy)
  calc_aero_coefficients/3(Cz) -> calc_aero_for_mom/6(Cz)
  calc_aero_coefficients/4(Cl) -> calc_aero_for_mom/7(Cl)
  calc_aero_coefficients/5(Cm) -> calc_aero_for_mom/8(Cm)
  calc_aero_coefficients/6(Cn) -> calc_aero_for_mom/9(Cn)
  Saturation1/1 -> calc_aero_coefficients/7(alB_deg)
  Saturation4/1 -> calc_aero_coefficients/8(beB_deg)
  Gain3/1 -> Saturation1/1
  Gain4/1 -> Saturation4/1

== system PIL_NO_RPI_new/Non-linear Flight Dynamic Model1/GRM_Airframe/aerodynamics/logic_base_drag ==
  env_glbl : Inport
  Bus Selector1 : BusSelector  OutputSignals=T_sim_glbl,T_sim_lnch
  Constant : Constant  Value=prp_T(end)
  MATLAB Function : MATLAB Function  TreatAsAtomicUnit=on
  Subtract : Sum  Inputs=+-
  flag_base_drag : Outport  VectorParamsAs1DForOutWhenUnconnected=off
  wires:
  Subtract/1 -> MATLAB Function/1(u)
  Constant/1 -> MATLAB Function/2(t_prp2)
  MATLAB Function/1(flag_base_drag) -> flag_base_drag/1  "flag_base_drag"
  Bus Selector1/1 -> Subtract/1  "<T_sim_glbl>"
  Bus Selector1/2 -> Subtract/2  "<T_sim_lnch>"
  env_glbl/1 -> Bus Selector1/1

== system PIL_NO_RPI_new/Non-linear Flight Dynamic Model1/GRM_Airframe/environment/WGS84_Gravitation ==
  lon : Inport  PortDimensions=1
  lat : Inport  Port=2  PortDimensions=1
  h : Inport  Port=3  PortDimensions=1
  Assertion : Assertion  AssertionFailFcn="error('WGS84 Gravitationsmodell: Die Werte des Eingangs \"h\" muessen groesser als 0 sein')"
  Assertion1 : Assertion  AssertionFailFcn="error('WGS84 Gravitationsmodell: Die Werte des Eingangs \"Long\" muessen zwischen -180 und +180 liegen')"
  Assertion2 : Assertion  AssertionFailFcn="error('WGS84 Gravitationsmodell: Die Werte des Eingangs \"Lat\" muessen zwischen -90 und +90 liegen')"
  Compare To Constant : simulink/Logic and Bit Operations/Compare To Constant  relop=>=  const=0  OutDataTypeStr=boolean
      settings: SourceProductName=ISim Simulink Block Set
  Interval Test : simulink/Logic and Bit Operations/Interval Test  IntervalClosedRight=on  uplimit=pi  IntervalClosedLeft=on  lowlimit=-pi  OutDataTypeStr=boolean
      settings: SourceProductName=ISim Simulink Block Set
  Interval Test1 : simulink/Logic and Bit Operations/Interval Test  IntervalClosedRight=on  uplimit=pi/2  IntervalClosedLeft=on  lowlimit=-pi/2  OutDataTypeStr=boolean
      settings: SourceProductName=ISim Simulink Block Set
  WGS84_2_ECEF : Subsystem
  WGS84_Gravity_Implementation : MATLAB Function  TreatAsAtomicUnit=on
  gE : Outport  PortDimensions=3  VectorParamsAs1DForOutWhenUnconnected=off
  wires:
  Interval Test1/1 -> Assertion2/1
  Interval Test/1 -> Assertion1/1
  Compare To Constant/1 -> Assertion/1
  WGS84_2_ECEF/1(pE) -> WGS84_Gravity_Implementation/1(pE)  "pE"
  lat/1 -> WGS84_Gravity_Implementation/2(lat_rad), Interval Test1/1, WGS84_2_ECEF/3(lat)  "lat"
  lon/1 -> WGS84_Gravity_Implementation/3(long_rad), Interval Test/1, WGS84_2_ECEF/2(lon)  "lon"
  h/1 -> WGS84_2_ECEF/1(h), Compare To Constant/1  "h"
  WGS84_Gravity_Implementation/1(gamma_R) -> gE/1  "gE"

== system PIL_NO_RPI_new/Non-linear Flight Dynamic Model1/GRM_Airframe/environment/atmosphere_static_ISO_2533 ==
  hBE : Inport
  env_glbl : Inport  Port=2
  Bus Creator1 : BusCreator  Inputs=6
  Bus Selector1 : BusSelector  OutputSignals=e_Tmp,e_pa
  Saturation : Saturate  UpperLimit=c_h_geope  LowerLimit=c_h_geop0
      settings: AttributesFormatString=|
      | %<UpperLimit>
      | %<LowerLimit>
  density : Subsystem
  geopot_height : Subsystem  mask{mean_earth_radius=c_r0}
      mask prompts: mean_earth_radius "Mean Earth Radius WGS 84 [m]"
      mask TypeOptions mean_earth_radius: mean_earth_radius/Value
  speed_of_sound : Subsystem
  tmp_and_pressure_ISO_2533 : Subsystem
  atm_stat : Outport  VectorParamsAs1DForOutWhenUnconnected=off
  wires:
  speed_of_sound/1(sos) -> Bus Creator1/3
  env_glbl/1 -> Bus Selector1/1
  Bus Selector1/2 -> tmp_and_pressure_ISO_2533/3(e_pa)  "<e_pa>"
  geopot_height/1(h_geop) -> Saturation/1
  Bus Selector1/1 -> tmp_and_pressure_ISO_2533/2(e_Tmp)  "<e_Tmp>"
  Bus Creator1/1 -> atm_stat/1  "atm_stat_bus"
  tmp_and_pressure_ISO_2533/1(Tmp) -> speed_of_sound/1(Tmp), Bus Creator1/4, density/1(Tmp)
  tmp_and_pressure_ISO_2533/2(pa) -> Bus Creator1/6, density/2(pa)
  density/1(rho) -> Bus Creator1/5
  hBE/1 -> Bus Creator1/1, geopot_height/1(hBE)
  Saturation/1 -> Bus Creator1/2, tmp_and_pressure_ISO_2533/1(h_geop)  "h_geop"

== system PIL_NO_RPI_new/Non-linear Flight Dynamic Model1/GRM_Airframe/environment/convert_to_local_frame ==
  gE : Inport
  Constant1 : Constant  Value=0
  Dot Product : DotProduct  InputSameDT=on  OutDataTypeStr=Inherit: Inherit via internal rule
  Sqrt : Sqrt  SaturateOnIntegerOverflow=on
  Vector Concatenate : Concatenate  NumInputs=3  Mode=Multidimensional array
  gBG : Outport  VectorParamsAs1DForOutWhenUnconnected=off
  wires:
  gE/1 -> Dot Product/1, Dot Product/2
  Constant1/1 -> Vector Concatenate/2, Vector Concatenate/1
  Sqrt/1 -> Vector Concatenate/3
  Vector Concatenate/1 -> gBG/1  "gBG"
  Dot Product/1 -> Sqrt/1

== system PIL_NO_RPI_new/Non-linear Flight Dynamic Model1/GRM_Airframe/fin_actuators/Rudder ==
  siB_c : Inport
  tRRR : Inport  Port=2
  Add : Sum  Inputs=+-
  Add1 : Sum  Inputs=+-
  Add2 : Sum  Inputs=+++
  Constant1 : Constant  Value=Actuator.fin1_bias
      settings: AttributesFormatString=%<Value>
  Gain : Gain  Gain=omega^2
  Gain2 : Gain  Gain=2*dmp*omega  Multiplication=Matrix(K*u)
  Gain3 : Gain  Gain=unc_bl
  Gain4 : Gain  Gain=Actuator.fin1_scale
      settings: AttributesFormatString=%<Gain>
  Integrator : Integrator  ExternalReset=either  InitialCondition=d_siB_0
  Integrator1 : Integrator  InitialCondition=siB_0  LimitOutput=on  UpperSaturationLimit=siB_max  LowerSaturationLimit=siB_min  ShowSaturationPort=on
  Limiting_Acceleration : MATLAB Function  TreatAsAtomicUnit=on
  Limiting_Rate : MATLAB Function  TreatAsAtomicUnit=on
  Saturation : Saturate  UpperLimit=siB_max  LowerLimit=siB_min
  Saturation1 : Saturate  UpperLimit=siB_max  LowerLimit=siB_min
  Sign : Signum
  siB : Outport  VectorParamsAs1DForOutWhenUnconnected=off
  d_siB : Outport  Port=2  VectorParamsAs1DForOutWhenUnconnected=off
  dd_siB : Outport  Port=3  VectorParamsAs1DForOutWhenUnconnected=off
  wires:
  Saturation1/1 -> siB/1, [siB]  "siB"
  Integrator1/2 -> Integrator/2  "sat"
  Gain4/1 -> Add2/2
  Gain3/1 -> Add2/3
  Sign/1 -> Gain3/1
  tRRR/1 -> Sign/1  "tRRR"
  Integrator1/1 -> Gain4/1, Add/2  "siB"
  Add1/1 -> Limiting_Acceleration/3(dd_siB)  "dd_siB"
  Gain2/1 -> Add1/2
  Gain/1 -> Add1/1
  Add/1 -> Gain/1
  Limiting_Acceleration/1(dd_siB_l) -> Integrator/1, dd_siB/1  "dd_siB_l"
  Limiting_Rate/1(d_siB_l) -> d_siB/1, [d_siB], Integrator1/1  "d_siB_l"
  Integrator/1 -> Limiting_Rate/2(d_siB), Gain2/1  "d_siB"
  Saturation/1 -> Add/1
  Add2/1 -> Saturation1/1
  Constant1/1 -> Add2/1
  siB_c/1 -> Saturation/1  "siB_c"
  [d_siB] -> Limiting_Acceleration/2(d_siB)
  [siB] -> Limiting_Acceleration/1(siB)
  [siB] -> Limiting_Rate/1(siB)

== system PIL_NO_RPI_new/Non-linear Flight Dynamic Model1/GRM_Airframe/fin_actuators/Rudder1 ==
  siB_c : Inport
  tRRR : Inport  Port=2
  Add : Sum  Inputs=+-
  Add1 : Sum  Inputs=+-
  Add3 : Sum  Inputs=+++
  Constant1 : Constant  Value=Actuator.fin2_bias
      settings: AttributesFormatString=%<Value>
  Gain : Gain  Gain=omega^2
  Gain2 : Gain  Gain=2*dmp*omega  Multiplication=Matrix(K*u)
  Gain3 : Gain  Gain=unc_bl
  Gain4 : Gain  Gain=Actuator.fin2_scale
      settings: AttributesFormatString=%<Gain>
  Integrator : Integrator  ExternalReset=either  InitialCondition=d_siB_0
  Integrator1 : Integrator  InitialCondition=siB_0  LimitOutput=on  UpperSaturationLimit=siB_max  LowerSaturationLimit=siB_min  ShowSaturationPort=on
  Limiting_Acceleration : MATLAB Function  TreatAsAtomicUnit=on
  Limiting_Rate : MATLAB Function  TreatAsAtomicUnit=on
  Saturation : Saturate  UpperLimit=siB_max  LowerLimit=siB_min
  Saturation1 : Saturate  UpperLimit=siB_max  LowerLimit=siB_min
  Sign : Signum
  siB : Outport  VectorParamsAs1DForOutWhenUnconnected=off
  d_siB : Outport  Port=2  VectorParamsAs1DForOutWhenUnconnected=off
  dd_siB : Outport  Port=3  VectorParamsAs1DForOutWhenUnconnected=off
  wires:
  Saturation1/1 -> siB/1, [siB]  "siB"
  Integrator1/2 -> Integrator/2  "sat"
  Gain3/1 -> Add3/3
  Sign/1 -> Gain3/1
  tRRR/1 -> Sign/1  "tRRR"
  Integrator1/1 -> Add/2, Gain4/1  "siB"
  Add1/1 -> Limiting_Acceleration/3(dd_siB)  "dd_siB"
  Gain2/1 -> Add1/2
  Gain/1 -> Add1/1
  Add/1 -> Gain/1
  Limiting_Acceleration/1(dd_siB_l) -> Integrator/1, dd_siB/1  "dd_siB_l"
  Limiting_Rate/1(d_siB_l) -> d_siB/1, [d_siB], Integrator1/1  "d_siB_l"
  Integrator/1 -> Limiting_Rate/2(d_siB), Gain2/1  "d_siB"
  Saturation/1 -> Add/1
  Add3/1 -> Saturation1/1
  siB_c/1 -> Saturation/1  "siB_c"
  [d_siB] -> Limiting_Acceleration/2(d_siB)
  [siB] -> Limiting_Acceleration/1(siB)
  [siB] -> Limiting_Rate/1(siB)
  Constant1/1 -> Add3/1
  Gain4/1 -> Add3/2

== system PIL_NO_RPI_new/Non-linear Flight Dynamic Model1/GRM_Airframe/fin_actuators/Rudder2 ==
  siB_c : Inport
  tRRR : Inport  Port=2
  Add : Sum  Inputs=+-
  Add1 : Sum  Inputs=+-
  Add3 : Sum  Inputs=+++
  Constant1 : Constant  Value=Actuator.fin3_bias
      settings: AttributesFormatString=%<Value>
  Gain : Gain  Gain=omega^2
  Gain2 : Gain  Gain=2*dmp*omega  Multiplication=Matrix(K*u)
  Gain3 : Gain  Gain=unc_bl
  Gain4 : Gain  Gain=Actuator.fin3_scale
      settings: AttributesFormatString=%<Gain>
  Integrator : Integrator  ExternalReset=either  InitialCondition=d_siB_0
  Integrator1 : Integrator  InitialCondition=siB_0  LimitOutput=on  UpperSaturationLimit=siB_max  LowerSaturationLimit=siB_min  ShowSaturationPort=on
  Limiting_Acceleration : MATLAB Function  TreatAsAtomicUnit=on
  Limiting_Rate : MATLAB Function  TreatAsAtomicUnit=on
  Saturation : Saturate  UpperLimit=siB_max  LowerLimit=siB_min
  Saturation1 : Saturate  UpperLimit=siB_max  LowerLimit=siB_min
  Sign : Signum
  siB : Outport  VectorParamsAs1DForOutWhenUnconnected=off
  d_siB : Outport  Port=2  VectorParamsAs1DForOutWhenUnconnected=off
  dd_siB : Outport  Port=3  VectorParamsAs1DForOutWhenUnconnected=off
  wires:
  Saturation1/1 -> siB/1, [siB]  "siB"
  Integrator1/2 -> Integrator/2  "sat"
  Gain3/1 -> Add3/3
  Sign/1 -> Gain3/1
  tRRR/1 -> Sign/1  "tRRR"
  Integrator1/1 -> Gain4/1, Add/2  "siB"
  Add1/1 -> Limiting_Acceleration/3(dd_siB)  "dd_siB"
  Gain2/1 -> Add1/2
  Gain/1 -> Add1/1
  Add/1 -> Gain/1
  Limiting_Acceleration/1(dd_siB_l) -> Integrator/1, dd_siB/1  "dd_siB_l"
  Limiting_Rate/1(d_siB_l) -> d_siB/1, [d_siB], Integrator1/1  "d_siB_l"
  Integrator/1 -> Limiting_Rate/2(d_siB), Gain2/1  "d_siB"
  Saturation/1 -> Add/1
  Add3/1 -> Saturation1/1
  siB_c/1 -> Saturation/1  "siB_c"
  [d_siB] -> Limiting_Acceleration/2(d_siB)
  [siB] -> Limiting_Acceleration/1(siB)
  [siB] -> Limiting_Rate/1(siB)
  Constant1/1 -> Add3/1
  Gain4/1 -> Add3/2
